simulink model "conversor_ADC"  (R2023b)
settings: Solver=VariableStepAuto  StartTime=0.0  StopTime=10.0  RelTol=1e-3
values from neighbouring files (symbols this model uses):
  Ts = interp_ts(Ts_ts,t)    [calcular_metricas_operacion.m]
libraries: simulink x5
settings Model: Creator=Pc  LastModifiedBy=Pc

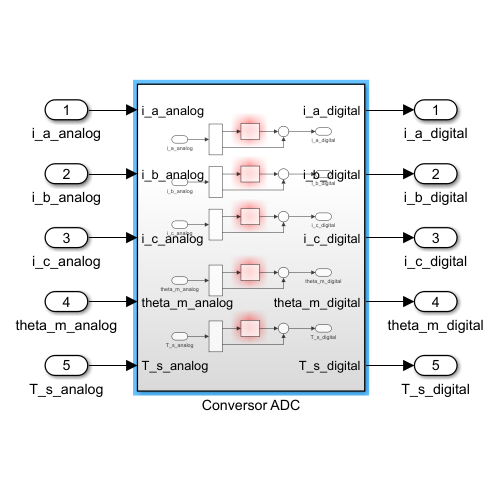
[thumbnail: Simulink's stored preview of the top-level diagram]
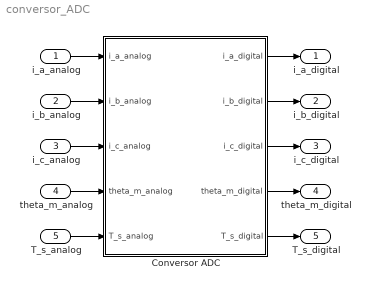
== system conversor_ADC ==
  i_a_analog : Inport
  i_b_analog : Inport  Port=2
  i_c_analog : Inport  Port=3
  theta_m_analog : Inport  Port=4
  T_s_analog : Inport  Port=5
  Conversor ADC : Subsystem
  i_a_digital : Outport
  i_b_digital : Outport  Port=2
  i_c_digital : Outport  Port=3
  theta_m_digital : Outport  Port=4
  T_s_digital : Outport  Port=5
  wires:
  i_a_analog/1 -> Conversor ADC/1(i_a_analog)
  i_b_analog/1 -> Conversor ADC/2(i_b_analog)
  i_c_analog/1 -> Conversor ADC/3(i_c_analog)
  theta_m_analog/1 -> Conversor ADC/4(theta_m_analog)
  T_s_analog/1 -> Conversor ADC/5(T_s_analog)
  Conversor ADC/1(i_a_digital) -> i_a_digital/1
  Conversor ADC/2(i_b_digital) -> i_b_digital/1
  Conversor ADC/3(i_c_digital) -> i_c_digital/1
  Conversor ADC/4(theta_m_digital) -> theta_m_digital/1
  Conversor ADC/5(T_s_digital) -> T_s_digital/1

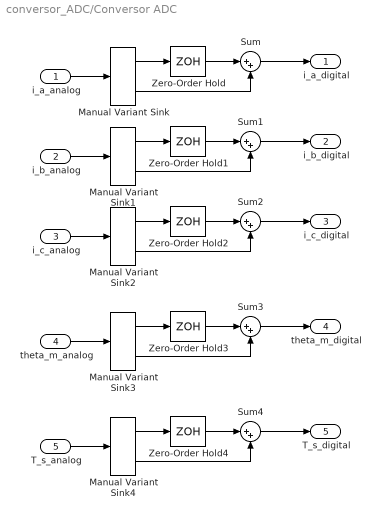
== system conversor_ADC/Conversor ADC ==
  i_a_analog : Inport
  i_b_analog : Inport  Port=2
  i_c_analog : Inport  Port=3
  theta_m_analog : Inport  Port=4
  T_s_analog : Inport  Port=5
  Manual Variant Sink{,1..4} (5 alike) : simulink/Signal Routing/Manual Variant Sink  NumChoices=2  LabelModeActiveChoice=V_2
  Sum{,1..4} (5 alike) : Sum  Inputs=|++
  Zero-Order Hold{,1..4} (5 alike) : ZeroOrderHold  SampleTime=Ts
  i_a_digital : Outport
  i_b_digital : Outport  Port=2
  i_c_digital : Outport  Port=3
  theta_m_digital : Outport  Port=4
  T_s_digital : Outport  Port=5
  wires:
  Zero-Order Hold1/1 -> Sum1/1
  theta_m_analog/1 -> Manual Variant Sink3/1
  Manual Variant Sink/2 -> Sum/2
  Manual Variant Sink3/2 -> Sum3/2
  Manual Variant Sink3/1 -> Zero-Order Hold3/1
  Manual Variant Sink/1 -> Zero-Order Hold/1
  Sum4/1 -> T_s_digital/1
  Sum2/1 -> i_c_digital/1
  i_a_analog/1 -> Manual Variant Sink/1
  Zero-Order Hold/1 -> Sum/1
  Manual Variant Sink1/1 -> Zero-Order Hold1/1
  Manual Variant Sink2/2 -> Sum2/2
  Sum1/1 -> i_b_digital/1
  Zero-Order Hold2/1 -> Sum2/1
  Zero-Order Hold3/1 -> Sum3/1
  Sum/1 -> i_a_digital/1
  Manual Variant Sink1/2 -> Sum1/2
  i_c_analog/1 -> Manual Variant Sink2/1
  Manual Variant Sink4/1 -> Zero-Order Hold4/1
  Zero-Order Hold4/1 -> Sum4/1
  i_b_analog/1 -> Manual Variant Sink1/1
  Manual Variant Sink4/2 -> Sum4/2
  T_s_analog/1 -> Manual Variant Sink4/1
  Manual Variant Sink2/1 -> Zero-Order Hold2/1
  Sum3/1 -> theta_m_digital/1
